simulink subsystem "Propulsion_Subsystem"  (R2026a)
settings: Solver=VariableStepAuto
settings Model: Creator=Eeman Aleem  LastModifiedBy=Eeman Aleem

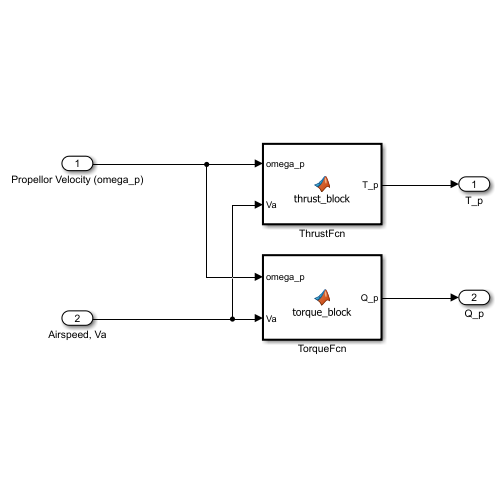
[thumbnail: Simulink's stored preview of the top-level diagram]
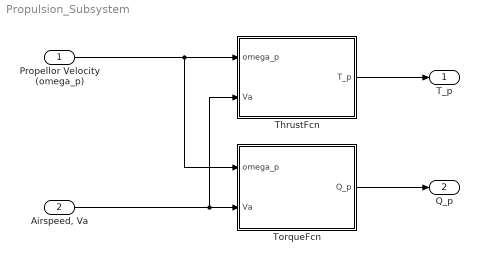
== system Propulsion_Subsystem ==
  Propellor Velocity (omega_p) : Inport
  "Airspeed, Va" : Inport  Port=2
  ThrustFcn : MATLAB Function  TreatAsAtomicUnit=on
  TorqueFcn : MATLAB Function  TreatAsAtomicUnit=on
  T_p : Outport
  Q_p : Outport  Port=2
  wires:
  ThrustFcn/1(T_p) -> T_p/1
  TorqueFcn/1(Q_p) -> Q_p/1
  Propellor Velocity (omega_p)/1 -> TorqueFcn/1(omega_p), ThrustFcn/1(omega_p)
  "Airspeed, Va"/1 -> ThrustFcn/2(Va), TorqueFcn/2(Va)

== matlab function Propulsion_Subsystem/ThrustFcn ==
  data: omega_p input; T_p output; Va input
function T_p = thrust_block(omega_p, Va)
rho = GeoConsts.rho; 
D = GeoConsts.D; 
k1 = LateralCoeffs.k1;
k2 = LateralCoeffs.k2;

if omega_p <= 0 || D <= 0
    J = 0; 
    C_T = 0;
else
    J = (2*pi*Va) / (omega_p*D);
    C_T = k1*J + k2*J^2;
end
T_p = [ ((rho*D^4/(4*pi^2)) * omega_p^2 * C_T) , 0, 0];
end

== matlab function Propulsion_Subsystem/TorqueFcn ==
  data: omega_p input; Q_p output; Va input
function Q_p = torque_block(omega_p, Va)
rho = GeoConsts.rho;
D = GeoConsts.D;
k1 = LateralCoeffs.k1;
k2 = LateralCoeffs.k2;

if omega_p <= 0 || D <= 0
    J = 0; 
    C_Q = 0;
else
    J = (2*pi*Va) / (omega_p*D);
    C_Q = k1*J + k2*J^2;
end
Q_p = [(rho*D^5/(4*pi^2)) * omega_p^2 * C_Q, 0, 0];
end
